simulink model "decimation"  (R2013b)
settings: Solver=ode45  StartTime=0.0  StopTime=10.0  RelTol=1e-3
undefined symbols (not defined in the file): xlfda_numerator
libraries: xbsIndex_r4 x1962, xps_library x2, casper_library_misc x1
(part 3 of 19)

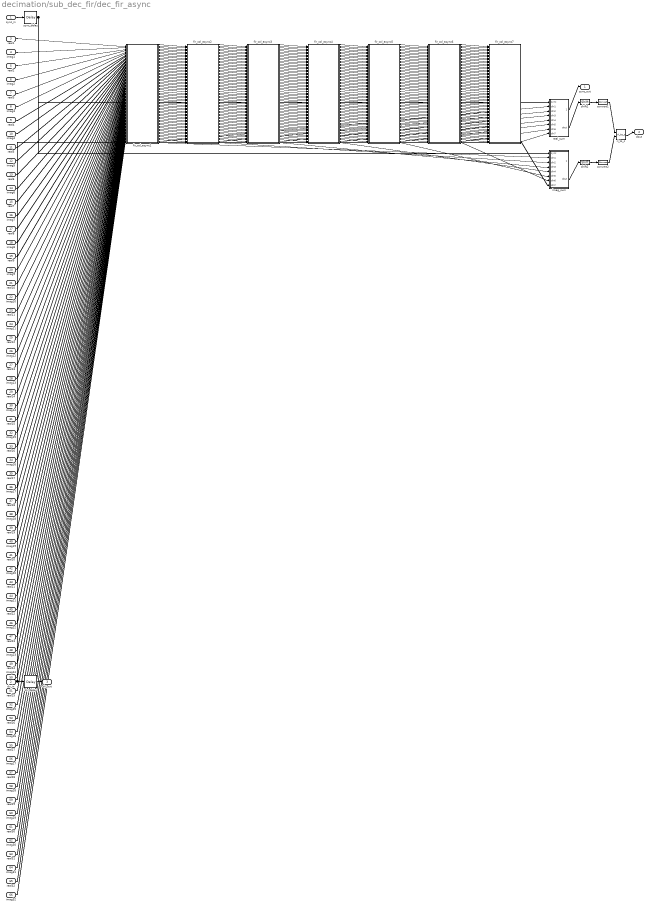
== system decimation/sub_dec_fir/dec_fir_async ==
  sync_in : Inport
  dv_in : Inport  Port=2
  real1 : Inport  Port=3
  imag1 : Inport  Port=4
  real2 : Inport  Port=5
  imag2 : Inport  Port=6
  real3 : Inport  Port=7
  imag3 : Inport  Port=8
  real4 : Inport  Port=9
  imag4 : Inport  Port=10
  real5 : Inport  Port=11
  imag5 : Inport  Port=12
  real6 : Inport  Port=13
  imag6 : Inport  Port=14
  real7 : Inport  Port=15
  imag7 : Inport  Port=16
  real8 : Inport  Port=17
  imag8 : Inport  Port=18
  real9 : Inport  Port=19
  imag9 : Inport  Port=20
  real10 : Inport  Port=21
  imag10 : Inport  Port=22
  real11 : Inport  Port=23
  imag11 : Inport  Port=24
  real12 : Inport  Port=25
  imag12 : Inport  Port=26
  real13 : Inport  Port=27
  imag13 : Inport  Port=28
  real14 : Inport  Port=29
  imag14 : Inport  Port=30
  real15 : Inport  Port=31
  imag15 : Inport  Port=32
  real16 : Inport  Port=33
  imag16 : Inport  Port=34
  real17 : Inport  Port=35
  imag17 : Inport  Port=36
  real18 : Inport  Port=37
  imag18 : Inport  Port=38
  real19 : Inport  Port=39
  imag19 : Inport  Port=40
  real20 : Inport  Port=41
  imag20 : Inport  Port=42
  real21 : Inport  Port=43
  imag21 : Inport  Port=44
  real22 : Inport  Port=45
  imag22 : Inport  Port=46
  real23 : Inport  Port=47
  imag23 : Inport  Port=48
  real24 : Inport  Port=49
  imag24 : Inport  Port=50
  real25 : Inport  Port=51
  imag25 : Inport  Port=52
  real26 : Inport  Port=53
  imag26 : Inport  Port=54
  real27 : Inport  Port=55
  imag27 : Inport  Port=56
  real28 : Inport  Port=57
  imag28 : Inport  Port=58
  real29 : Inport  Port=59
  imag29 : Inport  Port=60
  real30 : Inport  Port=61
  imag30 : Inport  Port=62
  real31 : Inport  Port=63
  imag31 : Inport  Port=64
  real32 : Inport  Port=65
  imag32 : Inport  Port=66
  convert1 : xbsIndex_r4/Convert  gui_display_data_type=Fixed-point  arith_type="Signed  (2's comp)"  n_bits=8  bin_pt=7  float_type=Single  exp_bits=8  fraction_bits=24  quantization="Round  (unbiased: +/- Inf)"  overflow=Wrap  en=off  latency=2  dbl_ovrd=off  pipeline=off  block_type=convert
  convert2 : xbsIndex_r4/Convert  gui_display_data_type=Fixed-point  arith_type="Signed  (2's comp)"  n_bits=8  bin_pt=7  float_type=Single  exp_bits=8  fraction_bits=24  quantization="Round  (unbiased: +/- Inf)"  overflow=Wrap  en=off  latency=2  dbl_ovrd=off  pipeline=off  block_type=convert
  dv_delay : xbsIndex_r4/Delay  rst=off  infoeditControl=Selection of Reset will increase slice count due to use of real FFs and instead of SRLs  en=off  latency=12  dbl_ovrd=off  reg_retiming=off  block_type=delay
  fir_col_async1 : Subsystem  AncestorBlock=casper_library_downconverter/fir_col_async  mask(fir_col_async){n_inputs=32, coeff=[2.094e-05  1.0782e-05 -1.2196e-05 -1.0656e-05  5.8959e-06  8.8553e-06 -1.8841e-06  -6.498e-06 -3.0314e-07  4.2696e-06  1.2212e-06 -2.5005e-06 -1.3767e-06  1.2723e-06  1.1591e-06 -5.2268e-07  -8.245e-07  1.2883e-07  5.1302e-07  3.7243e-08 -2.8089e-07  -7.936e-08  1.3374e-07  6.7875e-08 -5.3572e-08 -4.2603e-08  1.6753e-08  2.1193e-08 -3.3129e-09 -8.1838e-09  4.1399e-11  2.1483e-09], add_latency=1, mult_latency=2, coeff_bit_width=25, coeff_bin_pt=24, first_stage_hdl=on, adder_imp=DSP48, async=on, bus_input=off, input_width=0, input_bp=0, input_type=Signed, dbl=off}
      mask prompts: n_inputs "Inputs"; coeff "Coefficients"; add_latency "Add latency"; mult_latency "Mult Latency"; coeff_bit_width "Coefficient bit width"; coeff_bin_pt "Coefficient binary point"; first_stage_hdl "Implement first stage of adder trees on output as behavioural HDL"; adder_imp "Adder implementation"; async "Asynchronous ops"; bus_input "Bus input"; input_width "Input bitwidth"; input_bp "Input binary point"; input_type "Input datatype"; dbl "Double col"
      mask init:
      | fir_col_async_init(gcb);
      mask Help: eval('xlWeb(''http://casper.berkeley.edu/wiki/Fir_col'')')
      mask TypeOptions adder_imp: Behavioral | Fabric | DSP48
      mask Callback bus_input:
      | onoff = get_param(gcb, 'bus_input');
      | set_param_state(gcb, 'input_width', onoff)
      | set_param_state(gcb, 'input_bp', onoff)
      | set_param_state(gcb, 'input_type', onoff)
      mask TypeOptions input_type: Signed | Unsigned
  fir_col_async2 : Subsystem  AncestorBlock=casper_library_downconverter/fir_col_async  mask(fir_col_async){n_inputs=32, coeff=[-0.00038305   0.0009983  0.00059136 -0.00066133 -0.00066755  0.00035975  0.00064381 -0.00011772 -0.00055474 -5.5246e-05  0.00043232  0.00016117 -0.00030256 -0.00020986  0.00018397  0.00021522 -8.7435e-05 -0.00019207  1.7257e-05  0.00015386  2.7287e-05 -0.00011128 -5.0123e-05  7.1701e-05  5.6715e-05 -3.9326e-05 -5.2725e-05  1.5707e-05   4.312e-05 -5.1823e-07 -3.1693e-05 -7.6799e-06], add_latency=1, mult_latency=2, coeff_bit_width=25, coeff_bin_pt=24, first_stage_hdl=on, adder_imp=DSP48, async=on, bus_input=off, input_width=0, input_bp=0, input_type=Signed, dbl=off}
      mask prompts: n_inputs "Inputs"; coeff "Coefficients"; add_latency "Add latency"; mult_latency "Mult Latency"; coeff_bit_width "Coefficient bit width"; coeff_bin_pt "Coefficient binary point"; first_stage_hdl "Implement first stage of adder trees on output as behavioural HDL"; adder_imp "Adder implementation"; async "Asynchronous ops"; bus_input "Bus input"; input_width "Input bitwidth"; input_bp "Input binary point"; input_type "Input datatype"; dbl "Double col"
      mask init:
      | fir_col_async_init(gcb);
      mask Help: eval('xlWeb(''http://casper.berkeley.edu/wiki/Fir_col'')')
      mask TypeOptions adder_imp: Behavioral | Fabric | DSP48
      mask Callback bus_input:
      | onoff = get_param(gcb, 'bus_input');
      | set_param_state(gcb, 'input_width', onoff)
      | set_param_state(gcb, 'input_bp', onoff)
      | set_param_state(gcb, 'input_type', onoff)
      mask TypeOptions input_type: Signed | Unsigned
  fir_col_async3 : Subsystem  AncestorBlock=casper_library_downconverter/fir_col_async  mask(fir_col_async){n_inputs=32, coeff=[-0.015819  -0.0045283    0.012178   0.0072795  -0.0083697  -0.0085928    0.004768    0.008729  -0.0016445  -0.0079781  -0.0008307   0.0066367   0.0025836  -0.0049848  -0.0036243   0.0032652   0.0040292  -0.0016691  -0.0039196  0.00032909   0.0034399  0.00068177  -0.0027376  -0.0013435   0.0019468   0.0016792  -0.0011769  -0.0017418  0.00050609   0.0016008  1.9493e-05  -0.0013302], add_latency=1, mult_latency=2, coeff_bit_width=25, coeff_bin_pt=24, first_stage_hdl=on, adder_imp=DSP48, async=on, bus_input=off, input_width=0, input_bp=0, input_type=Signed, dbl=off}
      mask prompts: n_inputs "Inputs"; coeff "Coefficients"; add_latency "Add latency"; mult_latency "Mult Latency"; coeff_bit_width "Coefficient bit width"; coeff_bin_pt "Coefficient binary point"; first_stage_hdl "Implement first stage of adder trees on output as behavioural HDL"; adder_imp "Adder implementation"; async "Asynchronous ops"; bus_input "Bus input"; input_width "Input bitwidth"; input_bp "Input binary point"; input_type "Input datatype"; dbl "Double col"
      mask init:
      | fir_col_async_init(gcb);
      mask Help: eval('xlWeb(''http://casper.berkeley.edu/wiki/Fir_col'')')
      mask TypeOptions adder_imp: Behavioral | Fabric | DSP48
      mask Callback bus_input:
      | onoff = get_param(gcb, 'bus_input');
      | set_param_state(gcb, 'input_width', onoff)
      | set_param_state(gcb, 'input_bp', onoff)
      | set_param_state(gcb, 'input_type', onoff)
      mask TypeOptions input_type: Signed | Unsigned
  fir_col_async4 : Subsystem  AncestorBlock=casper_library_downconverter/fir_col_async  mask(fir_col_async){n_inputs=32, coeff=[0.00012251    0.018822   0.0061117   -0.020614   -0.014341    0.020479    0.024834   -0.017427   -0.038257   0.0097211    0.056618   0.0069114   -0.087351   -0.049861     0.17989     0.41449     0.41449     0.17989   -0.049861   -0.087351   0.0069114    0.056618   0.0097211   -0.038257   -0.017427    0.024834    0.020479   -0.014341   -0.020614   0.0061117    0.018822  0.00012251], add_latency=1, mult_latency=2, coeff_bit_width=25, coeff_bin_pt=24, first_stage_hdl=on, adder_imp=DSP48, async=on, bus_input=off, input_width=0, input_bp=0, input_type=Signed, dbl=off}
      mask prompts: n_inputs "Inputs"; coeff "Coefficients"; add_latency "Add latency"; mult_latency "Mult Latency"; coeff_bit_width "Coefficient bit width"; coeff_bin_pt "Coefficient binary point"; first_stage_hdl "Implement first stage of adder trees on output as behavioural HDL"; adder_imp "Adder implementation"; async "Asynchronous ops"; bus_input "Bus input"; input_width "Input bitwidth"; input_bp "Input binary point"; input_type "Input datatype"; dbl "Double col"
      mask init:
      | fir_col_async_init(gcb);
      mask Help: eval('xlWeb(''http://casper.berkeley.edu/wiki/Fir_col'')')
      mask TypeOptions adder_imp: Behavioral | Fabric | DSP48
      mask Callback bus_input:
      | onoff = get_param(gcb, 'bus_input');
      | set_param_state(gcb, 'input_width', onoff)
      | set_param_state(gcb, 'input_bp', onoff)
      | set_param_state(gcb, 'input_type', onoff)
      mask TypeOptions input_type: Signed | Unsigned
  fir_col_async5 : Subsystem  AncestorBlock=casper_library_downconverter/fir_col_async  mask(fir_col_async){n_inputs=32, coeff=[-0.0013302  1.9493e-05   0.0016008  0.00050609  -0.0017418  -0.0011769   0.0016792   0.0019468  -0.0013435  -0.0027376  0.00068177   0.0034399  0.00032909  -0.0039196  -0.0016691   0.0040292   0.0032652  -0.0036243  -0.0049848   0.0025836   0.0066367  -0.0008307  -0.0079781  -0.0016445    0.008729    0.004768  -0.0085928  -0.0083697   0.0072795    0.012178  -0.0045283   -0.015819], add_latency=1, mult_latency=2, coeff_bit_width=25, coeff_bin_pt=24, first_stage_hdl=on, adder_imp=DSP48, async=on, bus_input=off, input_width=0, input_bp=0, input_type=Signed, dbl=off}
      mask prompts: n_inputs "Inputs"; coeff "Coefficients"; add_latency "Add latency"; mult_latency "Mult Latency"; coeff_bit_width "Coefficient bit width"; coeff_bin_pt "Coefficient binary point"; first_stage_hdl "Implement first stage of adder trees on output as behavioural HDL"; adder_imp "Adder implementation"; async "Asynchronous ops"; bus_input "Bus input"; input_width "Input bitwidth"; input_bp "Input binary point"; input_type "Input datatype"; dbl "Double col"
      mask init:
      | fir_col_async_init(gcb);
      mask Help: eval('xlWeb(''http://casper.berkeley.edu/wiki/Fir_col'')')
      mask TypeOptions adder_imp: Behavioral | Fabric | DSP48
      mask Callback bus_input:
      | onoff = get_param(gcb, 'bus_input');
      | set_param_state(gcb, 'input_width', onoff)
      | set_param_state(gcb, 'input_bp', onoff)
      | set_param_state(gcb, 'input_type', onoff)
      mask TypeOptions input_type: Signed | Unsigned
  fir_col_async6 : Subsystem  AncestorBlock=casper_library_downconverter/fir_col_async  mask(fir_col_async){n_inputs=32, coeff=[-7.6799e-06 -3.1693e-05 -5.1823e-07   4.312e-05  1.5707e-05 -5.2725e-05 -3.9326e-05  5.6715e-05  7.1701e-05 -5.0123e-05 -0.00011128  2.7287e-05  0.00015386  1.7257e-05 -0.00019207 -8.7435e-05  0.00021522  0.00018397 -0.00020986 -0.00030256  0.00016117  0.00043232 -5.5246e-05 -0.00055474 -0.00011772  0.00064381  0.00035975 -0.00066755 -0.00066133  0.00059136   0.0009983 -0.00038305], add_latency=1, mult_latency=2, coeff_bit_width=25, coeff_bin_pt=24, first_stage_hdl=on, adder_imp=DSP48, async=on, bus_input=off, input_width=0, input_bp=0, input_type=Signed, dbl=off}
      mask prompts: n_inputs "Inputs"; coeff "Coefficients"; add_latency "Add latency"; mult_latency "Mult Latency"; coeff_bit_width "Coefficient bit width"; coeff_bin_pt "Coefficient binary point"; first_stage_hdl "Implement first stage of adder trees on output as behavioural HDL"; adder_imp "Adder implementation"; async "Asynchronous ops"; bus_input "Bus input"; input_width "Input bitwidth"; input_bp "Input binary point"; input_type "Input datatype"; dbl "Double col"
      mask init:
      | fir_col_async_init(gcb);
      mask Help: eval('xlWeb(''http://casper.berkeley.edu/wiki/Fir_col'')')
      mask TypeOptions adder_imp: Behavioral | Fabric | DSP48
      mask Callback bus_input:
      | onoff = get_param(gcb, 'bus_input');
      | set_param_state(gcb, 'input_width', onoff)
      | set_param_state(gcb, 'input_bp', onoff)
      | set_param_state(gcb, 'input_type', onoff)
      mask TypeOptions input_type: Signed | Unsigned
  fir_col_async7 : Subsystem  AncestorBlock=casper_library_downconverter/fir_col_async  mask(fir_col_async){n_inputs=32, coeff=[2.1483e-09  4.1399e-11 -8.1838e-09 -3.3129e-09  2.1193e-08  1.6753e-08 -4.2603e-08 -5.3572e-08  6.7875e-08  1.3374e-07  -7.936e-08 -2.8089e-07  3.7243e-08  5.1302e-07  1.2883e-07  -8.245e-07 -5.2268e-07  1.1591e-06  1.2723e-06 -1.3767e-06 -2.5005e-06  1.2212e-06  4.2696e-06 -3.0314e-07  -6.498e-06 -1.8841e-06  8.8553e-06  5.8959e-06 -1.0656e-05 -1.2196e-05  1.0782e-05   2.094e-05], add_latency=1, mult_latency=2, coeff_bit_width=25, coeff_bin_pt=24, first_stage_hdl=on, adder_imp=DSP48, async=on, bus_input=off, input_width=0, input_bp=0, input_type=Signed, dbl=off}
      mask prompts: n_inputs "Inputs"; coeff "Coefficients"; add_latency "Add latency"; mult_latency "Mult Latency"; coeff_bit_width "Coefficient bit width"; coeff_bin_pt "Coefficient binary point"; first_stage_hdl "Implement first stage of adder trees on output as behavioural HDL"; adder_imp "Adder implementation"; async "Asynchronous ops"; bus_input "Bus input"; input_width "Input bitwidth"; input_bp "Input binary point"; input_type "Input datatype"; dbl "Double col"
      mask init:
      | fir_col_async_init(gcb);
      mask Help: eval('xlWeb(''http://casper.berkeley.edu/wiki/Fir_col'')')
      mask TypeOptions adder_imp: Behavioral | Fabric | DSP48
      mask Callback bus_input:
      | onoff = get_param(gcb, 'bus_input');
      | set_param_state(gcb, 'input_width', onoff)
      | set_param_state(gcb, 'input_bp', onoff)
      | set_param_state(gcb, 'input_type', onoff)
      mask TypeOptions input_type: Signed | Unsigned
  imag_sum : Subsystem  AncestorBlock=casper_library_misc/adder_tree  mask(adder_tree){n_inputs=7, latency=1, adder_imp=DSP48, first_stage_hdl=off}
      mask prompts: n_inputs "Number of Inputs"; latency "Add Latency"; adder_imp "Adder implementation"; first_stage_hdl "Use behavioural HDL for first stage of adders"
      mask help:
      | Sums all inputs using a tree of adds and delays.
      |
      | Number of inputs: The number of inputs to the block to be summed
      | Add latency: The number of clock cycles to perform one addition (affects timing)..
      | Adder implementation: choice of fabric or DSP48E core, or behavioral HDL
      | Use behavioural HDL for first stage of adders: Causes the first stage of adders to be absorbed into DSP blocks if multipliers precede them (Virtex 5). Overrides Adder implementation
      mask init:
      | adder_tree_init(gcb, ...
      |     'n_inputs', n_inputs, ...
      |     'latency', latency, ...
      |     'adder_imp', adder_imp, ...
      |     'first_stage_hdl', first_stage_hdl);
      settings: AttributesFormatString=latency 3
      mask Help: eval('xlWeb(''http://casper.berkeley.edu/wiki/Adder_tree'')')
      mask TypeOptions adder_imp: Behavioral | Fabric | DSP48
  real_sum : Subsystem  AncestorBlock=casper_library_misc/adder_tree  mask(adder_tree){n_inputs=7, latency=1, adder_imp=DSP48, first_stage_hdl=off}
      mask prompts: n_inputs "Number of Inputs"; latency "Add Latency"; adder_imp "Adder implementation"; first_stage_hdl "Use behavioural HDL for first stage of adders"
      mask help:
      | Sums all inputs using a tree of adds and delays.
      |
      | Number of inputs: The number of inputs to the block to be summed
      | Add latency: The number of clock cycles to perform one addition (affects timing)..
      | Adder implementation: choice of fabric or DSP48E core, or behavioral HDL
      | Use behavioural HDL for first stage of adders: Causes the first stage of adders to be absorbed into DSP blocks if multipliers precede them (Virtex 5). Overrides Adder implementation
      mask init:
      | adder_tree_init(gcb, ...
      |     'n_inputs', n_inputs, ...
      |     'latency', latency, ...
      |     'adder_imp', adder_imp, ...
      |     'first_stage_hdl', first_stage_hdl);
      settings: AttributesFormatString=latency 3
      mask Help: eval('xlWeb(''http://casper.berkeley.edu/wiki/Adder_tree'')')
      mask TypeOptions adder_imp: Behavioral | Fabric | DSP48
  ri_to_c : casper_library_misc/ri_to_c
  shift1 : xbsIndex_r4/Shift  shift_dir=Left  shift_bits=1  en=off  latency=0  precision=Full  arith_type="Signed  (2's comp)"  n_bits=16  bin_pt=14  quantization=Truncate  overflow=Wrap  dbl_ovrd=off  block_type=shift
  shift2 : xbsIndex_r4/Shift  shift_dir=Left  shift_bits=1  en=off  latency=0  precision=Full  arith_type="Signed  (2's comp)"  n_bits=16  bin_pt=14  quantization=Truncate  overflow=Wrap  dbl_ovrd=off  block_type=shift
  sync_delay : xbsIndex_r4/Delay  rst=off  infoeditControl=Selection of Reset will increase slice count due to use of real FFs and instead of SRLs  en=off  latency=9  dbl_ovrd=off  reg_retiming=off  block_type=delay
  sync_out : Outport
  dout : Outport  Port=2
  dv_out : Outport  Port=3
  wires:
  sync_in/1 -> sync_delay/1
  dv_in/1 -> dv_delay/1, fir_col_async1/65(dv), fir_col_async2/65(dv), fir_col_async3/65(dv), fir_col_async4/65(dv), fir_col_async5/65(dv), fir_col_async6/65(dv), fir_col_async7/65(dv)
  dv_delay/1 -> dv_out/1
  real1/1 -> fir_col_async1/1(real1)
  imag1/1 -> fir_col_async1/2(imag1)
  real2/1 -> fir_col_async1/3(real2)
  imag2/1 -> fir_col_async1/4(imag2)
  real3/1 -> fir_col_async1/5(real3)
  imag3/1 -> fir_col_async1/6(imag3)
  real4/1 -> fir_col_async1/7(real4)
  imag4/1 -> fir_col_async1/8(imag4)
  real5/1 -> fir_col_async1/9(real5)
  imag5/1 -> fir_col_async1/10(imag5)
  real6/1 -> fir_col_async1/11(real6)
  imag6/1 -> fir_col_async1/12(imag6)
  real7/1 -> fir_col_async1/13(real7)
  imag7/1 -> fir_col_async1/14(imag7)
  real8/1 -> fir_col_async1/15(real8)
  imag8/1 -> fir_col_async1/16(imag8)
  real9/1 -> fir_col_async1/17(real9)
  imag9/1 -> fir_col_async1/18(imag9)
  real10/1 -> fir_col_async1/19(real10)
  imag10/1 -> fir_col_async1/20(imag10)
  real11/1 -> fir_col_async1/21(real11)
  imag11/1 -> fir_col_async1/22(imag11)
  real12/1 -> fir_col_async1/23(real12)
  imag12/1 -> fir_col_async1/24(imag12)
  real13/1 -> fir_col_async1/25(real13)
  imag13/1 -> fir_col_async1/26(imag13)
  real14/1 -> fir_col_async1/27(real14)
  imag14/1 -> fir_col_async1/28(imag14)
  real15/1 -> fir_col_async1/29(real15)
  imag15/1 -> fir_col_async1/30(imag15)
  real16/1 -> fir_col_async1/31(real16)
  imag16/1 -> fir_col_async1/32(imag16)
  real17/1 -> fir_col_async1/33(real17)
  imag17/1 -> fir_col_async1/34(imag17)
  real18/1 -> fir_col_async1/35(real18)
  imag18/1 -> fir_col_async1/36(imag18)
  real19/1 -> fir_col_async1/37(real19)
  imag19/1 -> fir_col_async1/38(imag19)
  real20/1 -> fir_col_async1/39(real20)
  imag20/1 -> fir_col_async1/40(imag20)
  real21/1 -> fir_col_async1/41(real21)
  imag21/1 -> fir_col_async1/42(imag21)
  real22/1 -> fir_col_async1/43(real22)
  imag22/1 -> fir_col_async1/44(imag22)
  real23/1 -> fir_col_async1/45(real23)
  imag23/1 -> fir_col_async1/46(imag23)
  real24/1 -> fir_col_async1/47(real24)
  imag24/1 -> fir_col_async1/48(imag24)
  real25/1 -> fir_col_async1/49(real25)
  imag25/1 -> fir_col_async1/50(imag25)
  real26/1 -> fir_col_async1/51(real26)
  imag26/1 -> fir_col_async1/52(imag26)
  real27/1 -> fir_col_async1/53(real27)
  imag27/1 -> fir_col_async1/54(imag27)
  real28/1 -> fir_col_async1/55(real28)
  imag28/1 -> fir_col_async1/56(imag28)
  real29/1 -> fir_col_async1/57(real29)
  imag29/1 -> fir_col_async1/58(imag29)
  real30/1 -> fir_col_async1/59(real30)
  imag30/1 -> fir_col_async1/60(imag30)
  real31/1 -> fir_col_async1/61(real31)
  imag31/1 -> fir_col_async1/62(imag31)
  real32/1 -> fir_col_async1/63(real32)
  imag32/1 -> fir_col_async1/64(imag32)
  fir_col_async1/65(real_sum) -> real_sum/2(din1)
  fir_col_async1/66(imag_sum) -> imag_sum/2(din1)
  fir_col_async1/1(real_out1) -> fir_col_async2/1(real1)
  fir_col_async1/2(imag_out1) -> fir_col_async2/2(imag1)
  fir_col_async1/3(real_out2) -> fir_col_async2/3(real2)
  fir_col_async1/4(imag_out2) -> fir_col_async2/4(imag2)
  fir_col_async1/5(real_out3) -> fir_col_async2/5(real3)
  fir_col_async1/6(imag_out3) -> fir_col_async2/6(imag3)
  fir_col_async1/7(real_out4) -> fir_col_async2/7(real4)
  fir_col_async1/8(imag_out4) -> fir_col_async2/8(imag4)
  fir_col_async1/9(real_out5) -> fir_col_async2/9(real5)
  fir_col_async1/10(imag_out5) -> fir_col_async2/10(imag5)
  fir_col_async1/11(real_out6) -> fir_col_async2/11(real6)
  fir_col_async1/12(imag_out6) -> fir_col_async2/12(imag6)
  fir_col_async1/13(real_out7) -> fir_col_async2/13(real7)
  fir_col_async1/14(imag_out7) -> fir_col_async2/14(imag7)
  fir_col_async1/15(real_out8) -> fir_col_async2/15(real8)
  fir_col_async1/16(imag_out8) -> fir_col_async2/16(imag8)
  fir_col_async1/17(real_out9) -> fir_col_async2/17(real9)
  fir_col_async1/18(imag_out9) -> fir_col_async2/18(imag9)
  fir_col_async1/19(real_out10) -> fir_col_async2/19(real10)
  fir_col_async1/20(imag_out10) -> fir_col_async2/20(imag10)
  fir_col_async1/21(real_out11) -> fir_col_async2/21(real11)
  fir_col_async1/22(imag_out11) -> fir_col_async2/22(imag11)
  fir_col_async1/23(real_out12) -> fir_col_async2/23(real12)
  fir_col_async1/24(imag_out12) -> fir_col_async2/24(imag12)
  fir_col_async1/25(real_out13) -> fir_col_async2/25(real13)
  fir_col_async1/26(imag_out13) -> fir_col_async2/26(imag13)
  fir_col_async1/27(real_out14) -> fir_col_async2/27(real14)
  fir_col_async1/28(imag_out14) -> fir_col_async2/28(imag14)
  fir_col_async1/29(real_out15) -> fir_col_async2/29(real15)
  fir_col_async1/30(imag_out15) -> fir_col_async2/30(imag15)
  fir_col_async1/31(real_out16) -> fir_col_async2/31(real16)
  fir_col_async1/32(imag_out16) -> fir_col_async2/32(imag16)
  fir_col_async1/33(real_out17) -> fir_col_async2/33(real17)
  fir_col_async1/34(imag_out17) -> fir_col_async2/34(imag17)
  fir_col_async1/35(real_out18) -> fir_col_async2/35(real18)
  fir_col_async1/36(imag_out18) -> fir_col_async2/36(imag18)
  fir_col_async1/37(real_out19) -> fir_col_async2/37(real19)
  fir_col_async1/38(imag_out19) -> fir_col_async2/38(imag19)
  fir_col_async1/39(real_out20) -> fir_col_async2/39(real20)
  fir_col_async1/40(imag_out20) -> fir_col_async2/40(imag20)
  fir_col_async1/41(real_out21) -> fir_col_async2/41(real21)
  fir_col_async1/42(imag_out21) -> fir_col_async2/42(imag21)
  fir_col_async1/43(real_out22) -> fir_col_async2/43(real22)
  fir_col_async1/44(imag_out22) -> fir_col_async2/44(imag22)
  fir_col_async1/45(real_out23) -> fir_col_async2/45(real23)
  fir_col_async1/46(imag_out23) -> fir_col_async2/46(imag23)
  fir_col_async1/47(real_out24) -> fir_col_async2/47(real24)
  fir_col_async1/48(imag_out24) -> fir_col_async2/48(imag24)
  fir_col_async1/49(real_out25) -> fir_col_async2/49(real25)
  fir_col_async1/50(imag_out25) -> fir_col_async2/50(imag25)
  fir_col_async1/51(real_out26) -> fir_col_async2/51(real26)
  fir_col_async1/52(imag_out26) -> fir_col_async2/52(imag26)
  fir_col_async1/53(real_out27) -> fir_col_async2/53(real27)
  fir_col_async1/54(imag_out27) -> fir_col_async2/54(imag27)
  fir_col_async1/55(real_out28) -> fir_col_async2/55(real28)
  fir_col_async1/56(imag_out28) -> fir_col_async2/56(imag28)
  fir_col_async1/57(real_out29) -> fir_col_async2/57(real29)
  fir_col_async1/58(imag_out29) -> fir_col_async2/58(imag29)
  fir_col_async1/59(real_out30) -> fir_col_async2/59(real30)
  fir_col_async1/60(imag_out30) -> fir_col_async2/60(imag30)
  fir_col_async1/61(real_out31) -> fir_col_async2/61(real31)
  fir_col_async1/62(imag_out31) -> fir_col_async2/62(imag31)
  fir_col_async1/63(real_out32) -> fir_col_async2/63(real32)
  fir_col_async1/64(imag_out32) -> fir_col_async2/64(imag32)
  fir_col_async2/65(real_sum) -> real_sum/3(din2)
  fir_col_async2/66(imag_sum) -> imag_sum/3(din2)
  fir_col_async2/1(real_out1) -> fir_col_async3/1(real1)
  fir_col_async2/2(imag_out1) -> fir_col_async3/2(imag1)
  fir_col_async2/3(real_out2) -> fir_col_async3/3(real2)
  fir_col_async2/4(imag_out2) -> fir_col_async3/4(imag2)
  fir_col_async2/5(real_out3) -> fir_col_async3/5(real3)
  fir_col_async2/6(imag_out3) -> fir_col_async3/6(imag3)
  fir_col_async2/7(real_out4) -> fir_col_async3/7(real4)
  fir_col_async2/8(imag_out4) -> fir_col_async3/8(imag4)
  fir_col_async2/9(real_out5) -> fir_col_async3/9(real5)
  fir_col_async2/10(imag_out5) -> fir_col_async3/10(imag5)
  fir_col_async2/11(real_out6) -> fir_col_async3/11(real6)
  fir_col_async2/12(imag_out6) -> fir_col_async3/12(imag6)
  fir_col_async2/13(real_out7) -> fir_col_async3/13(real7)
  fir_col_async2/14(imag_out7) -> fir_col_async3/14(imag7)
  fir_col_async2/15(real_out8) -> fir_col_async3/15(real8)
  fir_col_async2/16(imag_out8) -> fir_col_async3/16(imag8)
  fir_col_async2/17(real_out9) -> fir_col_async3/17(real9)
  fir_col_async2/18(imag_out9) -> fir_col_async3/18(imag9)
  fir_col_async2/19(real_out10) -> fir_col_async3/19(real10)
  fir_col_async2/20(imag_out10) -> fir_col_async3/20(imag10)
  fir_col_async2/21(real_out11) -> fir_col_async3/21(real11)
  fir_col_async2/22(imag_out11) -> fir_col_async3/22(imag11)
  fir_col_async2/23(real_out12) -> fir_col_async3/23(real12)
  fir_col_async2/24(imag_out12) -> fir_col_async3/24(imag12)
  fir_col_async2/25(real_out13) -> fir_col_async3/25(real13)
  fir_col_async2/26(imag_out13) -> fir_col_async3/26(imag13)
  fir_col_async2/27(real_out14) -> fir_col_async3/27(real14)
  fir_col_async2/28(imag_out14) -> fir_col_async3/28(imag14)
  fir_col_async2/29(real_out15) -> fir_col_async3/29(real15)
  fir_col_async2/30(imag_out15) -> fir_col_async3/30(imag15)
  fir_col_async2/31(real_out16) -> fir_col_async3/31(real16)
  fir_col_async2/32(imag_out16) -> fir_col_async3/32(imag16)
  fir_col_async2/33(real_out17) -> fir_col_async3/33(real17)
  fir_col_async2/34(imag_out17) -> fir_col_async3/34(imag17)
  fir_col_async2/35(real_out18) -> fir_col_async3/35(real18)
  fir_col_async2/36(imag_out18) -> fir_col_async3/36(imag18)
  fir_col_async2/37(real_out19) -> fir_col_async3/37(real19)
  fir_col_async2/38(imag_out19) -> fir_col_async3/38(imag19)
  fir_col_async2/39(real_out20) -> fir_col_async3/39(real20)
  fir_col_async2/40(imag_out20) -> fir_col_async3/40(imag20)
  fir_col_async2/41(real_out21) -> fir_col_async3/41(real21)
  fir_col_async2/42(imag_out21) -> fir_col_async3/42(imag21)
  fir_col_async2/43(real_out22) -> fir_col_async3/43(real22)
  fir_col_async2/44(imag_out22) -> fir_col_async3/44(imag22)
  fir_col_async2/45(real_out23) -> fir_col_async3/45(real23)
  fir_col_async2/46(imag_out23) -> fir_col_async3/46(imag23)
  fir_col_async2/47(real_out24) -> fir_col_async3/47(real24)
  fir_col_async2/48(imag_out24) -> fir_col_async3/48(imag24)
  fir_col_async2/49(real_out25) -> fir_col_async3/49(real25)
  fir_col_async2/50(imag_out25) -> fir_col_async3/50(imag25)
  fir_col_async2/51(real_out26) -> fir_col_async3/51(real26)
  fir_col_async2/52(imag_out26) -> fir_col_async3/52(imag26)
  fir_col_async2/53(real_out27) -> fir_col_async3/53(real27)
  fir_col_async2/54(imag_out27) -> fir_col_async3/54(imag27)
  fir_col_async2/55(real_out28) -> fir_col_async3/55(real28)
  fir_col_async2/56(imag_out28) -> fir_col_async3/56(imag28)
  fir_col_async2/57(real_out29) -> fir_col_async3/57(real29)
  fir_col_async2/58(imag_out29) -> fir_col_async3/58(imag29)
  fir_col_async2/59(real_out30) -> fir_col_async3/59(real30)
  fir_col_async2/60(imag_out30) -> fir_col_async3/60(imag30)
  fir_col_async2/61(real_out31) -> fir_col_async3/61(real31)
  fir_col_async2/62(imag_out31) -> fir_col_async3/62(imag31)
  fir_col_async2/63(real_out32) -> fir_col_async3/63(real32)
  fir_col_async2/64(imag_out32) -> fir_col_async3/64(imag32)
  fir_col_async3/65(real_sum) -> real_sum/4(din3)
  fir_col_async3/66(imag_sum) -> imag_sum/4(din3)
  fir_col_async3/1(real_out1) -> fir_col_async4/1(real1)
  fir_col_async3/2(imag_out1) -> fir_col_async4/2(imag1)
  fir_col_async3/3(real_out2) -> fir_col_async4/3(real2)
  fir_col_async3/4(imag_out2) -> fir_col_async4/4(imag2)
  fir_col_async3/5(real_out3) -> fir_col_async4/5(real3)
  fir_col_async3/6(imag_out3) -> fir_col_async4/6(imag3)
  fir_col_async3/7(real_out4) -> fir_col_async4/7(real4)
  fir_col_async3/8(imag_out4) -> fir_col_async4/8(imag4)
  fir_col_async3/9(real_out5) -> fir_col_async4/9(real5)
  fir_col_async3/10(imag_out5) -> fir_col_async4/10(imag5)
  fir_col_async3/11(real_out6) -> fir_col_async4/11(real6)
  fir_col_async3/12(imag_out6) -> fir_col_async4/12(imag6)
  fir_col_async3/13(real_out7) -> fir_col_async4/13(real7)
  fir_col_async3/14(imag_out7) -> fir_col_async4/14(imag7)
  fir_col_async3/15(real_out8) -> fir_col_async4/15(real8)
  fir_col_async3/16(imag_out8) -> fir_col_async4/16(imag8)
  fir_col_async3/17(real_out9) -> fir_col_async4/17(real9)
  fir_col_async3/18(imag_out9) -> fir_col_async4/18(imag9)
  fir_col_async3/19(real_out10) -> fir_col_async4/19(real10)
  fir_col_async3/20(imag_out10) -> fir_col_async4/20(imag10)
  fir_col_async3/21(real_out11) -> fir_col_async4/21(real11)
  fir_col_async3/22(imag_out11) -> fir_col_async4/22(imag11)
  fir_col_async3/23(real_out12) -> fir_col_async4/23(real12)
  fir_col_async3/24(imag_out12) -> fir_col_async4/24(imag12)
  fir_col_async3/25(real_out13) -> fir_col_async4/25(real13)
  fir_col_async3/26(imag_out13) -> fir_col_async4/26(imag13)
  fir_col_async3/27(real_out14) -> fir_col_async4/27(real14)
  fir_col_async3/28(imag_out14) -> fir_col_async4/28(imag14)
  fir_col_async3/29(real_out15) -> fir_col_async4/29(real15)
  fir_col_async3/30(imag_out15) -> fir_col_async4/30(imag15)
  fir_col_async3/31(real_out16) -> fir_col_async4/31(real16)
  fir_col_async3/32(imag_out16) -> fir_col_async4/32(imag16)
  fir_col_async3/33(real_out17) -> fir_col_async4/33(real17)
  fir_col_async3/34(imag_out17) -> fir_col_async4/34(imag17)
  fir_col_async3/35(real_out18) -> fir_col_async4/35(real18)
  fir_col_async3/36(imag_out18) -> fir_col_async4/36(imag18)
  fir_col_async3/37(real_out19) -> fir_col_async4/37(real19)
  fir_col_async3/38(imag_out19) -> fir_col_async4/38(imag19)
  fir_col_async3/39(real_out20) -> fir_col_async4/39(real20)
  fir_col_async3/40(imag_out20) -> fir_col_async4/40(imag20)
  fir_col_async3/41(real_out21) -> fir_col_async4/41(real21)
  fir_col_async3/42(imag_out21) -> fir_col_async4/42(imag21)
  fir_col_async3/43(real_out22) -> fir_col_async4/43(real22)
  fir_col_async3/44(imag_out22) -> fir_col_async4/44(imag22)
  fir_col_async3/45(real_out23) -> fir_col_async4/45(real23)
  fir_col_async3/46(imag_out23) -> fir_col_async4/46(imag23)
  fir_col_async3/47(real_out24) -> fir_col_async4/47(real24)
  fir_col_async3/48(imag_out24) -> fir_col_async4/48(imag24)
  fir_col_async3/49(real_out25) -> fir_col_async4/49(real25)
  fir_col_async3/50(imag_out25) -> fir_col_async4/50(imag25)
  fir_col_async3/51(real_out26) -> fir_col_async4/51(real26)
  fir_col_async3/52(imag_out26) -> fir_col_async4/52(imag26)
  fir_col_async3/53(real_out27) -> fir_col_async4/53(real27)
  fir_col_async3/54(imag_out27) -> fir_col_async4/54(imag27)
  fir_col_async3/55(real_out28) -> fir_col_async4/55(real28)
  fir_col_async3/56(imag_out28) -> fir_col_async4/56(imag28)
  fir_col_async3/57(real_out29) -> fir_col_async4/57(real29)
  fir_col_async3/58(imag_out29) -> fir_col_async4/58(imag29)
  fir_col_async3/59(real_out30) -> fir_col_async4/59(real30)
  fir_col_async3/60(imag_out30) -> fir_col_async4/60(imag30)
  fir_col_async3/61(real_out31) -> fir_col_async4/61(real31)
  fir_col_async3/62(imag_out31) -> fir_col_async4/62(imag31)
  fir_col_async3/63(real_out32) -> fir_col_async4/63(real32)
  fir_col_async3/64(imag_out32) -> fir_col_async4/64(imag32)
  fir_col_async4/65(real_sum) -> real_sum/5(din4)
  fir_col_async4/66(imag_sum) -> imag_sum/5(din4)
  fir_col_async4/1(real_out1) -> fir_col_async5/1(real1)
  fir_col_async4/2(imag_out1) -> fir_col_async5/2(imag1)
  fir_col_async4/3(real_out2) -> fir_col_async5/3(real2)
  fir_col_async4/4(imag_out2) -> fir_col_async5/4(imag2)
  fir_col_async4/5(real_out3) -> fir_col_async5/5(real3)
  fir_col_async4/6(imag_out3) -> fir_col_async5/6(imag3)
  fir_col_async4/7(real_out4) -> fir_col_async5/7(real4)
  fir_col_async4/8(imag_out4) -> fir_col_async5/8(imag4)
  fir_col_async4/9(real_out5) -> fir_col_async5/9(real5)
  fir_col_async4/10(imag_out5) -> fir_col_async5/10(imag5)
  fir_col_async4/11(real_out6) -> fir_col_async5/11(real6)
  fir_col_async4/12(imag_out6) -> fir_col_async5/12(imag6)
  fir_col_async4/13(real_out7) -> fir_col_async5/13(real7)
  fir_col_async4/14(imag_out7) -> fir_col_async5/14(imag7)
  fir_col_async4/15(real_out8) -> fir_col_async5/15(real8)
  fir_col_async4/16(imag_out8) -> fir_col_async5/16(imag8)
  fir_col_async4/17(real_out9) -> fir_col_async5/17(real9)
  fir_col_async4/18(imag_out9) -> fir_col_async5/18(imag9)
  fir_col_async4/19(real_out10) -> fir_col_async5/19(real10)
  fir_col_async4/20(imag_out10) -> fir_col_async5/20(imag10)
  fir_col_async4/21(real_out11) -> fir_col_async5/21(real11)
  fir_col_async4/22(imag_out11) -> fir_col_async5/22(imag11)
  fir_col_async4/23(real_out12) -> fir_col_async5/23(real12)
  fir_col_async4/24(imag_out12) -> fir_col_async5/24(imag12)
  fir_col_async4/25(real_out13) -> fir_col_async5/25(real13)
  fir_col_async4/26(imag_out13) -> fir_col_async5/26(imag13)
  fir_col_async4/27(real_out14) -> fir_col_async5/27(real14)
  fir_col_async4/28(imag_out14) -> fir_col_async5/28(imag14)
  fir_col_async4/29(real_out15) -> fir_col_async5/29(real15)
  fir_col_async4/30(imag_out15) -> fir_col_async5/30(imag15)
  fir_col_async4/31(real_out16) -> fir_col_async5/31(real16)
  fir_col_async4/32(imag_out16) -> fir_col_async5/32(imag16)
  fir_col_async4/33(real_out17) -> fir_col_async5/33(real17)
  fir_col_async4/34(imag_out17) -> fir_col_async5/34(imag17)
  fir_col_async4/35(real_out18) -> fir_col_async5/35(real18)
  fir_col_async4/36(imag_out18) -> fir_col_async5/36(imag18)
  fir_col_async4/37(real_out19) -> fir_col_async5/37(real19)
  fir_col_async4/38(imag_out19) -> fir_col_async5/38(imag19)
  fir_col_async4/39(real_out20) -> fir_col_async5/39(real20)
  fir_col_async4/40(imag_out20) -> fir_col_async5/40(imag20)
  fir_col_async4/41(real_out21) -> fir_col_async5/41(real21)
  fir_col_async4/42(imag_out21) -> fir_col_async5/42(imag21)
  fir_col_async4/43(real_out22) -> fir_col_async5/43(real22)
  fir_col_async4/44(imag_out22) -> fir_col_async5/44(imag22)
  fir_col_async4/45(real_out23) -> fir_col_async5/45(real23)
  fir_col_async4/46(imag_out23) -> fir_col_async5/46(imag23)
  fir_col_async4/47(real_out24) -> fir_col_async5/47(real24)
  fir_col_async4/48(imag_out24) -> fir_col_async5/48(imag24)
  fir_col_async4/49(real_out25) -> fir_col_async5/49(real25)
  fir_col_async4/50(imag_out25) -> fir_col_async5/50(imag25)
  fir_col_async4/51(real_out26) -> fir_col_async5/51(real26)
  fir_col_async4/52(imag_out26) -> fir_col_async5/52(imag26)
  fir_col_async4/53(real_out27) -> fir_col_async5/53(real27)
  fir_col_async4/54(imag_out27) -> fir_col_async5/54(imag27)
  fir_col_async4/55(real_out28) -> fir_col_async5/55(real28)
  fir_col_async4/56(imag_out28) -> fir_col_async5/56(imag28)
  fir_col_async4/57(real_out29) -> fir_col_async5/57(real29)
  fir_col_async4/58(imag_out29) -> fir_col_async5/58(imag29)
  fir_col_async4/59(real_out30) -> fir_col_async5/59(real30)
  fir_col_async4/60(imag_out30) -> fir_col_async5/60(imag30)
  fir_col_async4/61(real_out31) -> fir_col_async5/61(real31)
  fir_col_async4/62(imag_out31) -> fir_col_async5/62(imag31)
  fir_col_async4/63(real_out32) -> fir_col_async5/63(real32)
  fir_col_async4/64(imag_out32) -> fir_col_async5/64(imag32)
  fir_col_async5/65(real_sum) -> real_sum/6(din5)
  fir_col_async5/66(imag_sum) -> imag_sum/6(din5)
  fir_col_async5/1(real_out1) -> fir_col_async6/1(real1)
  fir_col_async5/2(imag_out1) -> fir_col_async6/2(imag1)
  fir_col_async5/3(real_out2) -> fir_col_async6/3(real2)
  fir_col_async5/4(imag_out2) -> fir_col_async6/4(imag2)
  fir_col_async5/5(real_out3) -> fir_col_async6/5(real3)
  fir_col_async5/6(imag_out3) -> fir_col_async6/6(imag3)
  fir_col_async5/7(real_out4) -> fir_col_async6/7(real4)
  fir_col_async5/8(imag_out4) -> fir_col_async6/8(imag4)
  fir_col_async5/9(real_out5) -> fir_col_async6/9(real5)
  fir_col_async5/10(imag_out5) -> fir_col_async6/10(imag5)
  fir_col_async5/11(real_out6) -> fir_col_async6/11(real6)
  fir_col_async5/12(imag_out6) -> fir_col_async6/12(imag6)
  fir_col_async5/13(real_out7) -> fir_col_async6/13(real7)
  fir_col_async5/14(imag_out7) -> fir_col_async6/14(imag7)
  fir_col_async5/15(real_out8) -> fir_col_async6/15(real8)
  fir_col_async5/16(imag_out8) -> fir_col_async6/16(imag8)
  fir_col_async5/17(real_out9) -> fir_col_async6/17(real9)
  fir_col_async5/18(imag_out9) -> fir_col_async6/18(imag9)
  fir_col_async5/19(real_out10) -> fir_col_async6/19(real10)
  fir_col_async5/20(imag_out10) -> fir_col_async6/20(imag10)
  fir_col_async5/21(real_out11) -> fir_col_async6/21(real11)
  fir_col_async5/22(imag_out11) -> fir_col_async6/22(imag11)
  fir_col_async5/23(real_out12) -> fir_col_async6/23(real12)
  fir_col_async5/24(imag_out12) -> fir_col_async6/24(imag12)
  fir_col_async5/25(real_out13) -> fir_col_async6/25(real13)
  fir_col_async5/26(imag_out13) -> fir_col_async6/26(imag13)
  fir_col_async5/27(real_out14) -> fir_col_async6/27(real14)
  fir_col_async5/28(imag_out14) -> fir_col_async6/28(imag14)
  fir_col_async5/29(real_out15) -> fir_col_async6/29(real15)
  fir_col_async5/30(imag_out15) -> fir_col_async6/30(imag15)
  fir_col_async5/31(real_out16) -> fir_col_async6/31(real16)
  fir_col_async5/32(imag_out16) -> fir_col_async6/32(imag16)
  fir_col_async5/33(real_out17) -> fir_col_async6/33(real17)
  fir_col_async5/34(imag_out17) -> fir_col_async6/34(imag17)
  fir_col_async5/35(real_out18) -> fir_col_async6/35(real18)
  fir_col_async5/36(imag_out18) -> fir_col_async6/36(imag18)
  fir_col_async5/37(real_out19) -> fir_col_async6/37(real19)
  fir_col_async5/38(imag_out19) -> fir_col_async6/38(imag19)
  fir_col_async5/39(real_out20) -> fir_col_async6/39(real20)
  fir_col_async5/40(imag_out20) -> fir_col_async6/40(imag20)
  fir_col_async5/41(real_out21) -> fir_col_async6/41(real21)
  fir_col_async5/42(imag_out21) -> fir_col_async6/42(imag21)
  fir_col_async5/43(real_out22) -> fir_col_async6/43(real22)
  fir_col_async5/44(imag_out22) -> fir_col_async6/44(imag22)
  fir_col_async5/45(real_out23) -> fir_col_async6/45(real23)
  fir_col_async5/46(imag_out23) -> fir_col_async6/46(imag23)
  fir_col_async5/47(real_out24) -> fir_col_async6/47(real24)
  fir_col_async5/48(imag_out24) -> fir_col_async6/48(imag24)
  fir_col_async5/49(real_out25) -> fir_col_async6/49(real25)
  fir_col_async5/50(imag_out25) -> fir_col_async6/50(imag25)
  fir_col_async5/51(real_out26) -> fir_col_async6/51(real26)
  fir_col_async5/52(imag_out26) -> fir_col_async6/52(imag26)
  fir_col_async5/53(real_out27) -> fir_col_async6/53(real27)
  fir_col_async5/54(imag_out27) -> fir_col_async6/54(imag27)
  fir_col_async5/55(real_out28) -> fir_col_async6/55(real28)
  fir_col_async5/56(imag_out28) -> fir_col_async6/56(imag28)
  fir_col_async5/57(real_out29) -> fir_col_async6/57(real29)
  fir_col_async5/58(imag_out29) -> fir_col_async6/58(imag29)
  fir_col_async5/59(real_out30) -> fir_col_async6/59(real30)
  fir_col_async5/60(imag_out30) -> fir_col_async6/60(imag30)
  fir_col_async5/61(real_out31) -> fir_col_async6/61(real31)
  fir_col_async5/62(imag_out31) -> fir_col_async6/62(imag31)
  fir_col_async5/63(real_out32) -> fir_col_async6/63(real32)
  fir_col_async5/64(imag_out32) -> fir_col_async6/64(imag32)
  fir_col_async6/65(real_sum) -> real_sum/7(din6)
  fir_col_async6/66(imag_sum) -> imag_sum/7(din6)
  fir_col_async6/1(real_out1) -> fir_col_async7/1(real1)
  fir_col_async6/2(imag_out1) -> fir_col_async7/2(imag1)
  fir_col_async6/3(real_out2) -> fir_col_async7/3(real2)
  fir_col_async6/4(imag_out2) -> fir_col_async7/4(imag2)
  fir_col_async6/5(real_out3) -> fir_col_async7/5(real3)
  fir_col_async6/6(imag_out3) -> fir_col_async7/6(imag3)
  fir_col_async6/7(real_out4) -> fir_col_async7/7(real4)
  fir_col_async6/8(imag_out4) -> fir_col_async7/8(imag4)
  fir_col_async6/9(real_out5) -> fir_col_async7/9(real5)
  fir_col_async6/10(imag_out5) -> fir_col_async7/10(imag5)
  fir_col_async6/11(real_out6) -> fir_col_async7/11(real6)
  fir_col_async6/12(imag_out6) -> fir_col_async7/12(imag6)
  fir_col_async6/13(real_out7) -> fir_col_async7/13(real7)
  fir_col_async6/14(imag_out7) -> fir_col_async7/14(imag7)
  fir_col_async6/15(real_out8) -> fir_col_async7/15(real8)
  fir_col_async6/16(imag_out8) -> fir_col_async7/16(imag8)
  fir_col_async6/17(real_out9) -> fir_col_async7/17(real9)
  fir_col_async6/18(imag_out9) -> fir_col_async7/18(imag9)
  fir_col_async6/19(real_out10) -> fir_col_async7/19(real10)
  fir_col_async6/20(imag_out10) -> fir_col_async7/20(imag10)
  fir_col_async6/21(real_out11) -> fir_col_async7/21(real11)
  fir_col_async6/22(imag_out11) -> fir_col_async7/22(imag11)
  fir_col_async6/23(real_out12) -> fir_col_async7/23(real12)
  fir_col_async6/24(imag_out12) -> fir_col_async7/24(imag12)
  fir_col_async6/25(real_out13) -> fir_col_async7/25(real13)
  fir_col_async6/26(imag_out13) -> fir_col_async7/26(imag13)
  fir_col_async6/27(real_out14) -> fir_col_async7/27(real14)
  fir_col_async6/28(imag_out14) -> fir_col_async7/28(imag14)
  fir_col_async6/29(real_out15) -> fir_col_async7/29(real15)
  fir_col_async6/30(imag_out15) -> fir_col_async7/30(imag15)
  fir_col_async6/31(real_out16) -> fir_col_async7/31(real16)
  fir_col_async6/32(imag_out16) -> fir_col_async7/32(imag16)
  fir_col_async6/33(real_out17) -> fir_col_async7/33(real17)
  fir_col_async6/34(imag_out17) -> fir_col_async7/34(imag17)
  fir_col_async6/35(real_out18) -> fir_col_async7/35(real18)
  fir_col_async6/36(imag_out18) -> fir_col_async7/36(imag18)
  fir_col_async6/37(real_out19) -> fir_col_async7/37(real19)
  fir_col_async6/38(imag_out19) -> fir_col_async7/38(imag19)
  fir_col_async6/39(real_out20) -> fir_col_async7/39(real20)
  fir_col_async6/40(imag_out20) -> fir_col_async7/40(imag20)
  fir_col_async6/41(real_out21) -> fir_col_async7/41(real21)
  fir_col_async6/42(imag_out21) -> fir_col_async7/42(imag21)
  fir_col_async6/43(real_out22) -> fir_col_async7/43(real22)
  fir_col_async6/44(imag_out22) -> fir_col_async7/44(imag22)
  fir_col_async6/45(real_out23) -> fir_col_async7/45(real23)
  fir_col_async6/46(imag_out23) -> fir_col_async7/46(imag23)
  fir_col_async6/47(real_out24) -> fir_col_async7/47(real24)
  fir_col_async6/48(imag_out24) -> fir_col_async7/48(imag24)
  fir_col_async6/49(real_out25) -> fir_col_async7/49(real25)
  fir_col_async6/50(imag_out25) -> fir_col_async7/50(imag25)
  fir_col_async6/51(real_out26) -> fir_col_async7/51(real26)
  fir_col_async6/52(imag_out26) -> fir_col_async7/52(imag26)
  fir_col_async6/53(real_out27) -> fir_col_async7/53(real27)
  fir_col_async6/54(imag_out27) -> fir_col_async7/54(imag27)
  fir_col_async6/55(real_out28) -> fir_col_async7/55(real28)
  fir_col_async6/56(imag_out28) -> fir_col_async7/56(imag28)
  fir_col_async6/57(real_out29) -> fir_col_async7/57(real29)
  fir_col_async6/58(imag_out29) -> fir_col_async7/58(imag29)
  fir_col_async6/59(real_out30) -> fir_col_async7/59(real30)
  fir_col_async6/60(imag_out30) -> fir_col_async7/60(imag30)
  fir_col_async6/61(real_out31) -> fir_col_async7/61(real31)
  fir_col_async6/62(imag_out31) -> fir_col_async7/62(imag31)
  fir_col_async6/63(real_out32) -> fir_col_async7/63(real32)
  fir_col_async6/64(imag_out32) -> fir_col_async7/64(imag32)
  fir_col_async7/65(real_sum) -> real_sum/8(din7)
  fir_col_async7/66(imag_sum) -> imag_sum/8(din7)
  real_sum/2(dout) -> shift1/1
  imag_sum/2(dout) -> shift2/1
  shift1/1 -> convert1/1
  shift2/1 -> convert2/1
  convert1/1 -> ri_to_c/1
  convert2/1 -> ri_to_c/2
  ri_to_c/1 -> dout/1
  sync_delay/1 -> real_sum/1(sync), imag_sum/1(sync)
  real_sum/1(sync_out) -> sync_out/1
